simulink model "rekonstr_1"  (Simulink 7.7)
settings: Solver=ode45  StartTime=0.0  StopTime=5.0  RelTol=1e-3
values from neighbouring files (symbols this model uses):
  frausch = 250    [analog_bp3.m]    (also in analog_tp2.m = 500)
  fs = 16000    [G722_1.m]    (also in TP_fdesign1.m = 0.215; adaptiv_2.m = 1000; adaptiv_3.m = 1000; adaptiv_4.m = 1000)
  h = firpm(64,f,m)    [CFIR_1.m]    (also in adapt_filter1.m = adaptfilt.lms(ni,mu); adapt_filter2.m = adaptfilt.blms(ni,mu,1,36); adaptiv_2.m = [1 2 3 4 5 6 7 8 9 10]; adaptiv_3.m = [1 2 3 4 5 6 7 8 9 10])
libraries: dsparch4 x3
settings Model: Creator=svenhoffmann  LastModifiedBy=josef  ExtModeAutoUpdateStatusClock=off
settings DataIOCC: MaxDataPoints=5000  SignalLoggingName=sigsOut  OutputOption=SpecifiedOutputTimes  OutputTimes=[0:1e-4:5]
settings DebuggingCC: SaveWithParameterizedLinksMsg=none  SignalResolutionControl=TryResolveAllWithWarning  SolverPrmCheckMsg=none  MultiTaskDSMMsg=warning  MultiTaskCondExecSysMsg=none  StrictBusMsg=None
settings HardwareCC: TargetUnknown=on
settings RTWCC: IncludeERTFirstTime=on

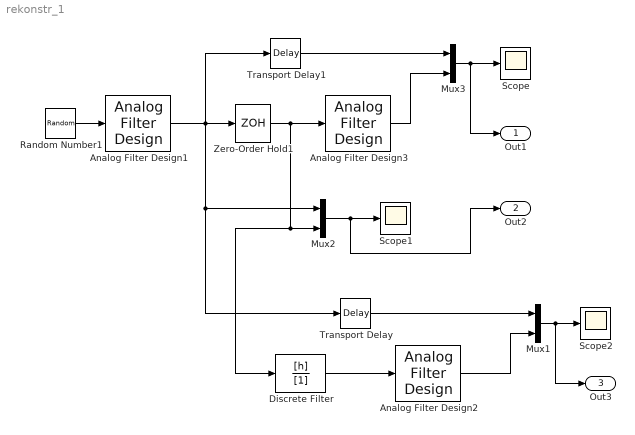
== system rekonstr_1 ==
  Analog Filter Design1 : dsparch4/Analog Filter Design  method=Chebyshev I  filttype=Lowpass  N=8  Wlo=2*pi*frausch  Whi=80  Rp=2  Rs=40
  Analog Filter Design2 : dsparch4/Analog Filter Design  method=Butterworth  filttype=Lowpass  N=8  Wlo=2*pi*fs/2  Whi=80  Rp=2  Rs=40
  Analog Filter Design3 : dsparch4/Analog Filter Design  method=Butterworth  filttype=Lowpass  N=8  Wlo=2*pi*fs/2  Whi=80  Rp=2  Rs=40
  Discrete Filter : DiscreteFilter  Numerator=[h]  Denominator=[1]  SampleTime=1/fs
  Mux1 : Mux  Inputs=2
  Mux2 : Mux  Inputs=2
  Mux3 : Mux  Inputs=2
  Random Number1 : RandomNumber  Seed=13790  SampleTime=0
  Scope : Scope
  Scope1 : Scope
  Scope2 : Scope
      settings: SaveName=ScopeData2
  Transport Delay : TransportDelay  DelayTime=3.25e-3
  Transport Delay1 : TransportDelay  DelayTime=2.2e-3
  Zero-Order Hold1 : ZeroOrderHold  SampleTime=1/fs
  Out1 : Outport
  Out2 : Outport  Port=2
  Out3 : Outport  Port=3
  wires:
  Mux1/1 -> Out3/1, Scope2/1
  Transport Delay/1 -> Mux1/1
  Analog Filter Design2/1 -> Mux1/2
  Random Number1/1 -> Analog Filter Design1/1
  Analog Filter Design1/1 -> Transport Delay1/1, Zero-Order Hold1/1, Mux2/1, Transport Delay/1
  Zero-Order Hold1/1 -> Analog Filter Design3/1, Mux2/2, Discrete Filter/1
  Mux2/1 -> Out2/1, Scope1/1
  Mux3/1 -> Out1/1, Scope/1
  Transport Delay1/1 -> Mux3/1
  Analog Filter Design3/1 -> Mux3/2
  Discrete Filter/1 -> Analog Filter Design2/1
